simulink model "zadaca1Simulink"  (R2018a)
settings: Solver=VariableStepAuto  StartTime=0.0  StopTime=20  RelTol=1e-3
settings Model: Creator=User  LastModifiedBy=User

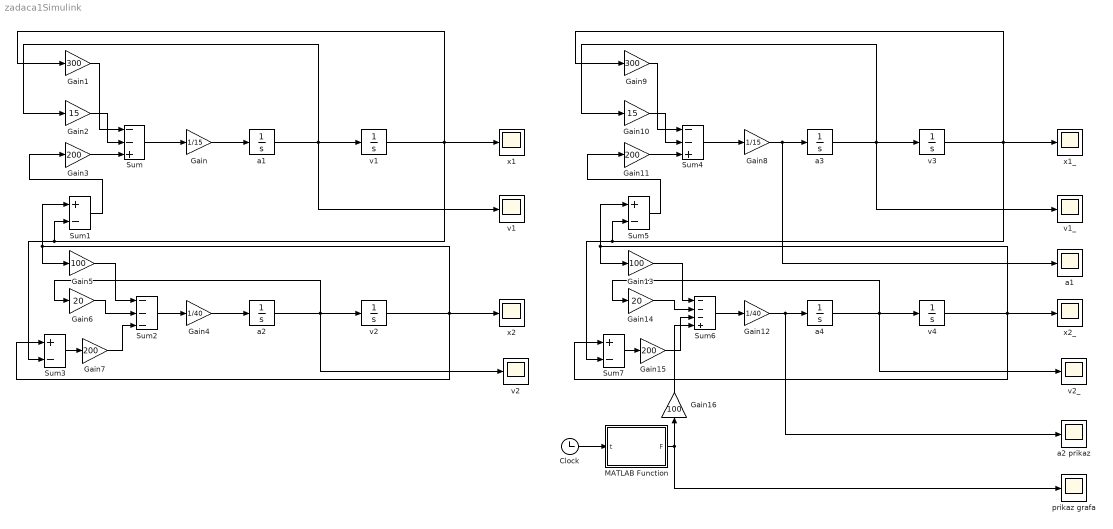
== system zadaca1Simulink ==
  Clock : Clock
  Gain : Gain  Gain=1/15
  Gain1 : Gain  Gain=300
  Gain10 : Gain  Gain=15
  Gain{3,7,11,15} (4 alike) : Gain  Gain=200
  Gain12 : Gain  Gain=1/40
  Gain13 : Gain  Gain=100
  Gain14 : Gain  Gain=20
  Gain16 : Gain  Gain=100
  Gain2 : Gain  Gain=15
  Gain4 : Gain  Gain=1/40
  Gain5 : Gain  Gain=100
  Gain6 : Gain  Gain=20
  Gain8 : Gain  Gain=1/15
  Gain9 : Gain  Gain=300
  MATLAB Function : MATLAB Function  TreatAsAtomicUnit=on
  Sum : Sum  Inputs=--+
  Sum{1,3,5,7} (4 alike) : Sum  Inputs=+-
  Sum2 : Sum  Inputs=---
  Sum4 : Sum  Inputs=--+
  Sum6 : Sum  Inputs=---+
  a{1..4} (4 alike) : Integrator
  "a1 " : Scope
  a2 prikaz : Scope
  prikaz grafa : Scope
  v1 : Integrator  InitialCondition=5
  "v1 " : Scope
  v1_ : Scope
  v2 : Integrator
  "v2 " : Scope
  "v2_ " : Scope
  v3 : Integrator
  v4 : Integrator
  x1 : Scope
  x1_ : Scope
  x2 : Scope
  "x2_ " : Scope
  wires:
  a1/1 -> v1/1, "v1 "/1, Gain2/1
  v1/1 -> Sum1/2, Sum3/2, Gain1/1, x1/1
  Gain/1 -> a1/1
  Sum/1 -> Gain/1
  Sum1/1 -> Gain3/1
  Gain3/1 -> Sum/3
  Gain2/1 -> Sum/2
  Gain1/1 -> Sum/1
  v2/1 -> Sum3/1, Sum1/1, Gain5/1, x2/1
  a2/1 -> "v2 "/1, Gain6/1, v2/1
  Gain4/1 -> a2/1
  Sum2/1 -> Gain4/1
  Gain5/1 -> Sum2/1
  Gain6/1 -> Sum2/2
  Sum3/1 -> Gain7/1
  Gain7/1 -> Sum2/3
  Gain11/1 -> Sum4/3
  Gain9/1 -> Sum4/1
  Gain10/1 -> Sum4/2
  Sum5/1 -> Gain11/1
  v3/1 -> Sum5/2, Sum7/2, Gain9/1, x1_/1
  Gain14/1 -> Sum6/2
  a3/1 -> v3/1, v1_/1, Gain10/1
  a4/1 -> "v2_ "/1, Gain14/1, v4/1
  Sum6/1 -> Gain12/1
  Gain12/1 -> a2 prikaz/1, a4/1
  Gain8/1 -> "a1 "/1, a3/1
  Gain13/1 -> Sum6/1
  Sum4/1 -> Gain8/1
  v4/1 -> Sum7/1, Sum5/1, Gain13/1, "x2_ "/1
  Sum7/1 -> Gain15/1
  Gain15/1 -> Sum6/3
  Clock/1 -> MATLAB Function/1(t)
  MATLAB Function/1(F) -> Gain16/1, prikaz grafa/1
  Gain16/1 -> Sum6/4

== matlab function zadaca1Simulink/MATLAB Function ==
  data: t input; F output
function F = ForceF(t)
% F = ForceF(t)
    F = zeros(size(t)); % Initialize the output F to have the same size as t
    for i = 1:length(t)
        time = t(i);
        time_mod = mod(time, 4);
        if time_mod >= 0 && time_mod < 1
            F(i) = time_mod;
        elseif time_mod >= 1 && time_mod < 2
            F(i) = -time_mod + 2;
        elseif time_mod == 2
            F(i) = 2;
        elseif time_mod > 2 && time_mod <= 3
            F(i) = time_mod;
        elseif time_mod >= 3 && time_mod < 4
            F(i) = -time_mod+6;
        elseif time_mod == 4
            F(i) = 0;
        end
    end
end
